simulink model "adaptativeControl"  (R2023b)
settings: Solver=VariableStepAuto  StartTime=0.0  StopTime=time(end)  FixedStep=10e-17  RelTol=1e-3
undefined symbols (not defined in the file): DiscIntNeverNeededParam
libraries: simulink x1
settings Model: Creator=v4pal  LastModifiedBy=v4pal

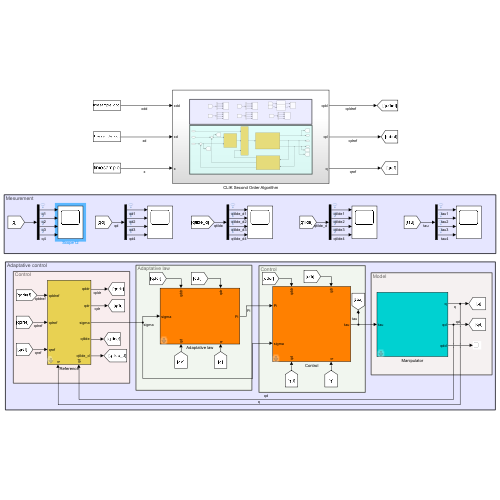
[thumbnail: Simulink's stored preview of the top-level diagram]
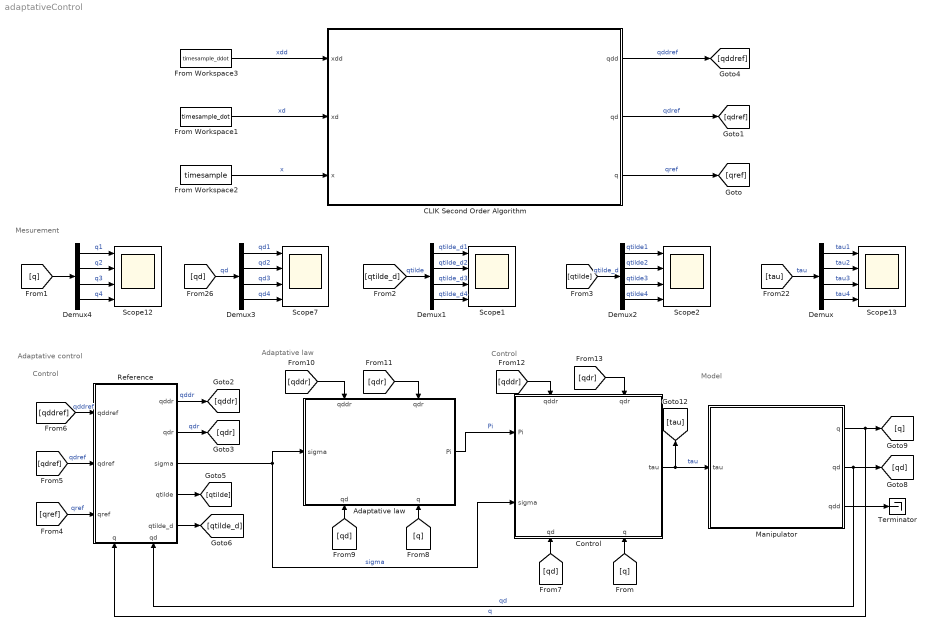
== system adaptativeControl ==
  note: Control
  note: Adaptative law
  note: Mesurement
  note: Control
  note: Adaptative control
  note: Model
  Adaptative law : Subsystem  mask{Kpi=50000}
      mask prompts: Kpi "K_PI"
      settings: PortSchema="{\"entries\":[{\"content\":{\"sides\":[{\"content\":{\"connectorIds\":[\"In1\"]},\"type\":\"ConnectorPlacement.EquallySpacedRectSide\",\"uuid\":\"db15ee83-1f1b-455d-afda-e94c97dcc1f2\"},{\"content\":{\"connectorIds\":[\"Out1\"],\"side\":\"RIGHT\"},\"type\":\"ConnectorPlacement.EquallySpacedRectSide\",\"uuid\":\"41c3f407-56b1-4c5a-b932-c27e17c703ed\"},{\"content\":{\"connectorIds\":[\"In2\",\"In3\"],\"side\":\"TOP\"},\"type\":\"ConnectorPlacement.EquallySpacedRectSide\",\"uuid\":\"e06182f5-78d8-4c0d-9fb3-4a5678e4fb72\"},{\"content\":{\"connectorIds\":[\"In4\",\"In5\"],\"side\":\"BOTTOM\"},\"type\":\"ConnectorPlacement.EquallySpacedRectSide\",\"uuid\":\"7434239a-7bad-433a-9a5d-3d00bbee33a9\"}]},\"type\":\"ConnectorPlacement.EquallySpacedConnector\",\"uuid\":\"7980dd28-bdab-4e8b-a843-8afbd90a57e5\"}],\"packageUris\":[\"http://schema.mathworks.com/mf0/Connector/R2020b\"],\"version\":\"1.0\"}"
  CLIK Second Order Algorithm : Subsystem
  Control : Subsystem  mask{Kd=300}
      settings: PortSchema="{\"entries\":[{\"content\":{\"sides\":[{\"content\":{\"connectorIds\":[\"In1\",\"In2\"]},\"type\":\"ConnectorPlacement.EquallySpacedRectSide\",\"uuid\":\"acb7cdf1-642f-4969-8ed4-672da436f71d\"},{\"content\":{\"connectorIds\":[\"Out1\"],\"side\":\"RIGHT\"},\"type\":\"ConnectorPlacement.EquallySpacedRectSide\",\"uuid\":\"4cc46839-d0fa-4cc4-8f70-8a289b8a20bb\"},{\"content\":{\"connectorIds\":[\"In3\",\"In4\"],\"side\":\"TOP\"},\"type\":\"ConnectorPlacement.EquallySpacedRectSide\",\"uuid\":\"a17c3f60-f42b-40f7-9d43-81c6c657e972\"},{\"content\":{\"connectorIds\":[\"In5\",\"In6\"],\"side\":\"BOTTOM\"},\"type\":\"ConnectorPlacement.EquallySpacedRectSide\",\"uuid\":\"3f3a44a0-a063-4d17-9e5f-328f3f6552e7\"}]},\"type\":\"ConnectorPlacement.EquallySpacedConnector\",\"uuid\":\"f4f2dfd8-ded6-4248-b856-2003e9c40e79\"}],\"packageUris\":[\"http://schema.mathworks.com/mf0/Connector/R2020b\"],\"version\":\"1.0\"}"
  Demux{,1..4} (5 alike) : Demux
  From Workspace1 : FromWorkspace  VariableName=timesample_dot
  From Workspace2 : FromWorkspace  VariableName=timesample
  From Workspace3 : FromWorkspace  VariableName=timesample_ddot
  Manipulator : Subsystem  mask{m_load=4, delta=10}
      mask prompts: m_load "Load Mass [kg]"; delta "Uncertainty [%]"
      mask DialogControl DescGroupVar Prompt: SCARA Dynamic Model
      mask DialogControl DescTextVar Prompt: Scara Dynamic Model with uncertainty and load mass as input.
  Reference : Subsystem  mask{lambda=10}
      settings: PortSchema="{\"entries\":[{\"content\":{\"sides\":[{\"content\":{\"connectorIds\":[\"In1\",\"In2\",\"In3\"]},\"type\":\"ConnectorPlacement.EquallySpacedRectSide\",\"uuid\":\"cb63d9dc-23a2-4ec7-ac11-e398610ef5c2\"},{\"content\":{\"connectorIds\":[\"Out1\",\"Out2\",\"Out3\",\"Out4\",\"Out5\"],\"side\":\"RIGHT\"},\"type\":\"ConnectorPlacement.EquallySpacedRectSide\",\"uuid\":\"29d086a8-0031-4faa-9200-b9934d21fc49\"},{\"content\":{\"side\":\"TOP\"},\"type\":\"ConnectorPlacement.EquallySpacedRectSide\",\"uuid\":\"49ce7692-caef-46fe-903f-68a05e9f5245\"},{\"content\":{\"connectorIds\":[\"In4\",\"In5\"],\"side\":\"BOTTOM\"},\"type\":\"ConnectorPlacement.EquallySpacedRectSide\",\"uuid\":\"32e605e3-ac7e-458a-bf29-966abc0750c1\"}]},\"type\":\"ConnectorPlacement.EquallySpacedConnector\",\"uuid\":\"b951568f-fc90-455a-8420-9594f5316c31\"}],\"packageUris\":[\"http://schema.mathworks.com/mf0/Connector/R2020b\"],\"version\":\"1.0\"}"
  Scope{1..2,7,12..13} (5 alike) : Scope  NumInputPorts=4
  Terminator : Terminator
  wires:
  [qd] -> Demux3/1  "qd"
  Demux2/2 -> Scope2/2  "qtilde2"
  Demux2/3 -> Scope2/3  "qtilde3"
  Demux2/4 -> Scope2/4  "qtilde4"
  [q] -> Demux4/1
  Demux4/4 -> Scope12/4  "q4"
  [qtilde] -> Demux2/1  "qtilde_d"
  Demux1/2 -> Scope1/2  "qtilde_d2"
  Demux1/4 -> Scope1/4  "qtilde_d4"
  [qtilde_d] -> Demux1/1  "qtilde"
  Demux3/4 -> Scope7/4  "qd4"
  Demux3/3 -> Scope7/3  "qd3"
  Demux3/2 -> Scope7/2  "qd2"
  Demux1/1 -> Scope1/1  "qtilde_d1"
  Demux3/1 -> Scope7/1  "qd1"
  Demux/3 -> Scope13/3  "tau3"
  Manipulator/2(qd) -> Reference/5(qd), [qd]  "qd"
  Demux/2 -> Scope13/2  "tau2"
  Control/1(tau) -> Manipulator/1(tau), [tau]  "tau"
  Demux2/1 -> Scope2/1  "qtilde1"
  Demux1/3 -> Scope1/3  "qtilde_d3"
  Demux4/1 -> Scope12/1  "q1"
  Demux/4 -> Scope13/4  "tau4"
  [tau] -> Demux/1  "tau"
  Demux/1 -> Scope13/1  "tau1"
  Demux4/3 -> Scope12/3  "q3"
  Manipulator/3(qdd) -> Terminator/1
  Demux4/2 -> Scope12/2  "q2"
  Manipulator/1(q) -> Reference/4(q), [q]  "q"
  [qddref] -> Reference/1(qddref)  "qddref"
  [qdref] -> Reference/2(qdref)  "qdref"
  [qref] -> Reference/3(qref)  "qref"
  Adaptative law/1(Pi) -> Control/1(Pi)  "Pi"
  Reference/3(sigma) -> Control/2(sigma), Adaptative law/1(sigma)  "sigma"
  [q] -> Control/6(q)
  [qd] -> Control/5(qd)
  [q] -> Adaptative law/5(q)
  [qd] -> Adaptative law/4(qd)
  Reference/1(qddr) -> [qddr]  "qddr"
  Reference/2(qdr) -> [qdr]  "qdr"
  [qddr] -> Adaptative law/2(qddr)
  [qdr] -> Adaptative law/3(qdr)
  [qddr] -> Control/3(qddr)
  [qdr] -> Control/4(qdr)
  Reference/4(qtilde) -> [qtilde]
  Reference/5(qtilde_d) -> [qtilde_d]
  CLIK Second Order Algorithm/2(qd) -> [qdref]  "qdref"
  CLIK Second Order Algorithm/1(qdd) -> [qddref]  "qddref"
  CLIK Second Order Algorithm/3(q) -> [qref]  "qref"
  From Workspace1/1 -> CLIK Second Order Algorithm/2(xd)  "xd"
  From Workspace3/1 -> CLIK Second Order Algorithm/1(xdd)  "xdd"
  From Workspace2/1 -> CLIK Second Order Algorithm/3(x)  "x"

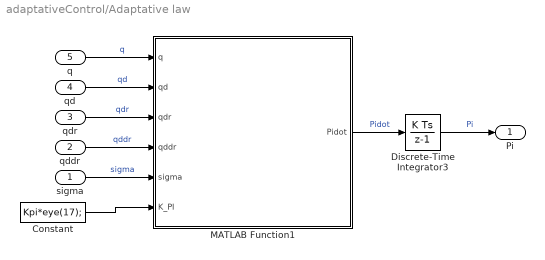
== system adaptativeControl/Adaptative law ==
  sigma : Inport
  qddr : Inport  Port=2
  qdr : Inport  Port=3
  qd : Inport  Port=4
  q : Inport  Port=5
  Constant : Constant  Value=Kpi*eye(17);
  Discrete-Time Integrator3 : DiscreteIntegrator  InitialCondition=[1.2500, 20.0000, 5.0000, 1.2500, 10.0000, 4, 4.000, 4.0000, 1.0000, 0.0100, 0.0100, 0.0050, 0.0010, 0.0001, 0.0001, 0.0100, 0.0050]'  SampleTime=0.001  ICPrevOutput=DiscIntNeverNeededParam  ICPrevScaledInput=DiscIntNeverNeededParam
  MATLAB Function1 : MATLAB Function  TreatAsAtomicUnit=on
  Pi : Outport
  wires:
  q/1 -> MATLAB Function1/1(q)  "q"
  MATLAB Function1/1(Pidot) -> Discrete-Time Integrator3/1  "Pidot"
  Discrete-Time Integrator3/1 -> Pi/1  "Pi"
  qd/1 -> MATLAB Function1/2(qd)  "qd"
  qdr/1 -> MATLAB Function1/3(qdr)  "qdr"
  sigma/1 -> MATLAB Function1/5(sigma)  "sigma"
  qddr/1 -> MATLAB Function1/4(qddr)  "qddr"
  Constant/1 -> MATLAB Function1/6(K_PI)

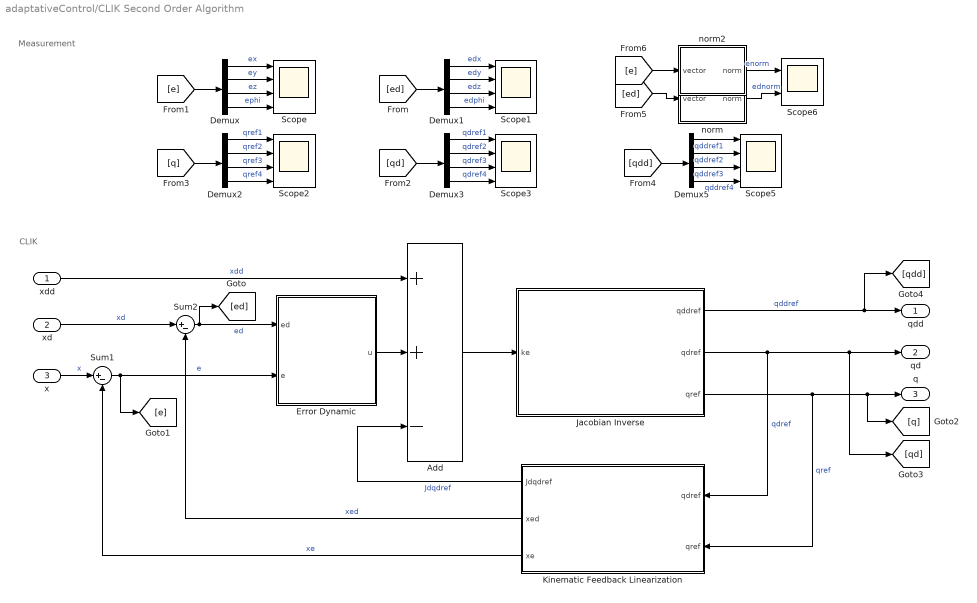
== system adaptativeControl/CLIK Second Order Algorithm ==
  note: CLIK
  note: Measurement
  xdd : Inport
  xd : Inport  Port=2
  x : Inport  Port=3
  Add : Sum  Inputs=++-
  Demux{,1..3,5} (5 alike) : Demux
  Error Dynamic : Subsystem  mask{Kd1=10, Kd2=10, Kd3=10, Kd4=10, Kp1=500, Kp2=500, Kp3=500, Kp4=500, Ki=0}
  Jacobian Inverse : Subsystem
  Kinematic Feedback Linearization : Subsystem
  Scope{,1..3,5} (5 alike) : Scope  NumInputPorts=4
  Scope6 : Scope  NumInputPorts=2
  Sum1 : Sum  Inputs=|+-
  Sum2 : Sum  Inputs=|+-
  norm : Subsystem
  norm2 : Subsystem
  qdd : Outport
  qd : Outport  Port=2
  q : Outport  Port=3
  wires:
  Sum1/1 -> Error Dynamic/2(e), [e]  "e"
  Jacobian Inverse/2(qdref) -> [qd], qd/1, Kinematic Feedback Linearization/1(qdref)  "qdref"
  Sum2/1 -> Error Dynamic/1(ed), [ed]  "ed"
  Add/1 -> Jacobian Inverse/1(ke)
  x/1 -> Sum1/1  "x"
  Jacobian Inverse/3(qref) -> [q], q/1, Kinematic Feedback Linearization/2(qref)  "qref"
  Kinematic Feedback Linearization/1(Jdqdref) -> Add/3  "Jdqdref"
  Kinematic Feedback Linearization/3(xe) -> Sum1/2  "xe"
  Kinematic Feedback Linearization/2(xed) -> Sum2/2  "xed"
  xd/1 -> Sum2/1  "xd"
  Jacobian Inverse/1(qddref) -> [qdd], qdd/1  "qddref"
  xdd/1 -> Add/1  "xdd"
  [ed] -> Demux1/1
  [e] -> Demux/1
  Demux/1 -> Scope/1  "ex"
  Demux/2 -> Scope/2  "ey"
  Demux/3 -> Scope/3  "ez"
  Demux/4 -> Scope/4  "ephi"
  Demux1/1 -> Scope1/1  "edx"
  Demux1/2 -> Scope1/2  "edy"
  Demux1/3 -> Scope1/3  "edz"
  Demux1/4 -> Scope1/4  "edphi"
  Demux3/4 -> Scope3/4  "qdref4"
  Demux3/3 -> Scope3/3  "qdref3"
  Demux3/2 -> Scope3/2  "qdref2"
  Demux3/1 -> Scope3/1  "qdref1"
  Demux2/4 -> Scope2/4  "qref4"
  Demux2/3 -> Scope2/3  "qref3"
  Demux2/2 -> Scope2/2  "qref2"
  Demux2/1 -> Scope2/1  "qref1"
  [q] -> Demux2/1
  [qd] -> Demux3/1
  [qdd] -> Demux5/1
  Demux5/1 -> Scope5/1  "qddref1"
  Demux5/2 -> Scope5/2  "qddref2"
  Demux5/3 -> Scope5/3  "qddref3"
  Demux5/4 -> Scope5/4  "qddref4"
  [e] -> norm2/1(vector)
  norm2/1(norm) -> Scope6/1  "enorm"
  norm/1(norm) -> Scope6/2  "ednorm"
  [ed] -> norm/1(vector)
  Error Dynamic/1(u) -> Add/2

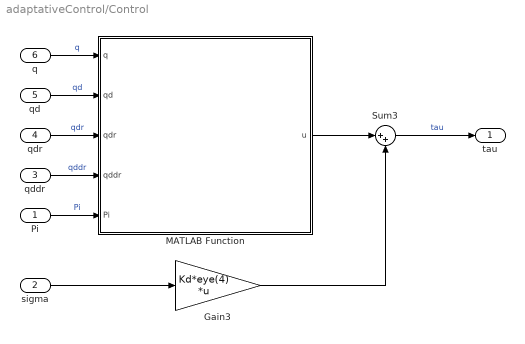
== system adaptativeControl/Control ==
  Pi : Inport
  sigma : Inport  Port=2
  qddr : Inport  Port=3
  qdr : Inport  Port=4
  qd : Inport  Port=5
  q : Inport  Port=6
  Gain3 : Gain  Gain=Kd*eye(4)  Multiplication=Matrix(K*u)
  MATLAB Function : MATLAB Function  TreatAsAtomicUnit=on
  Sum3 : Sum  Inputs=|++
  tau : Outport
  wires:
  Gain3/1 -> Sum3/2
  qd/1 -> MATLAB Function/2(qd)  "qd"
  Pi/1 -> MATLAB Function/5(Pi)  "Pi"
  MATLAB Function/1(u) -> Sum3/1
  Sum3/1 -> tau/1  "tau"
  q/1 -> MATLAB Function/1(q)  "q"
  qdr/1 -> MATLAB Function/3(qdr)  "qdr"
  qddr/1 -> MATLAB Function/4(qddr)  "qddr"
  sigma/1 -> Gain3/1

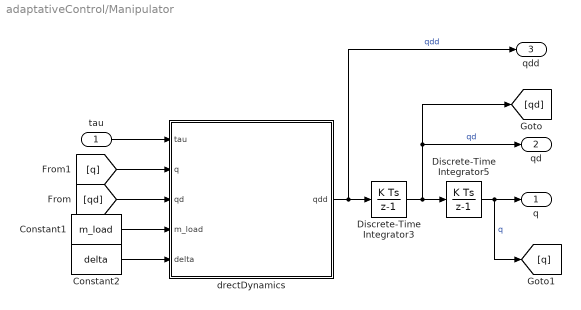
== system adaptativeControl/Manipulator ==
  tau : Inport
  Constant1 : Constant  Value=m_load
  Constant2 : Constant  Value=delta
  Discrete-Time Integrator3 : DiscreteIntegrator  InitialCondition=[0; 0; 0; 0]  SampleTime=0.001  ICPrevOutput=DiscIntNeverNeededParam  ICPrevScaledInput=DiscIntNeverNeededParam
  Discrete-Time Integrator5 : DiscreteIntegrator  InitialCondition=[-1.5706; 0.7851; 0.5000; -0.7855]  SampleTime=0.001  ICPrevOutput=DiscIntNeverNeededParam  ICPrevScaledInput=DiscIntNeverNeededParam
  drectDynamics : MATLAB Function  TreatAsAtomicUnit=on
  q : Outport
  qd : Outport  Port=2
  qdd : Outport  Port=3
  wires:
  tau/1 -> drectDynamics/1(tau)
  Constant1/1 -> drectDynamics/4(m_load)
  drectDynamics/1(qdd) -> qdd/1, Discrete-Time Integrator3/1  "qdd"
  Discrete-Time Integrator3/1 -> [qd], qd/1, Discrete-Time Integrator5/1  "qd"
  Discrete-Time Integrator5/1 -> [q], q/1  "q"
  [qd] -> drectDynamics/3(qd)
  [q] -> drectDynamics/2(q)
  Constant2/1 -> drectDynamics/5(delta)

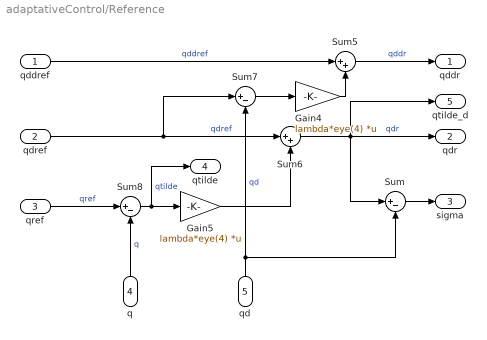
== system adaptativeControl/Reference ==
  qddref : Inport
  qdref : Inport  Port=2
  qref : Inport  Port=3
  q : Inport  Port=4
  qd : Inport  Port=5
  Gain4 : Gain  Gain=lambda*eye(4)  Multiplication=Matrix(K*u)
  Gain5 : Gain  Gain=lambda*eye(4)  Multiplication=Matrix(K*u)
  Sum : Sum  Inputs=|+-
  Sum5 : Sum  Inputs=|++
  Sum6 : Sum  Inputs=|++
  Sum7 : Sum  Inputs=|+-
  Sum8 : Sum  Inputs=|+-
  qddr : Outport
  qdr : Outport  Port=2
  sigma : Outport  Port=3
  qtilde : Outport  Port=4
  qtilde_d : Outport  Port=5
  wires:
  qdref/1 -> Sum7/1, Sum6/1  "qdref"
  Sum8/1 -> qtilde/1, Gain5/1  "qtilde"
  Sum6/1 -> qtilde_d/1, Sum/1, qdr/1  "qdr"
  Gain5/1 -> Sum6/2
  q/1 -> Sum8/2  "q"
  Gain4/1 -> Sum5/2
  Sum7/1 -> Gain4/1
  Sum5/1 -> qddr/1  "qddr"
  qref/1 -> Sum8/1  "qref"
  qddref/1 -> Sum5/1  "qddref"
  qd/1 -> Sum/2, Sum7/2  "qd"
  Sum/1 -> sigma/1

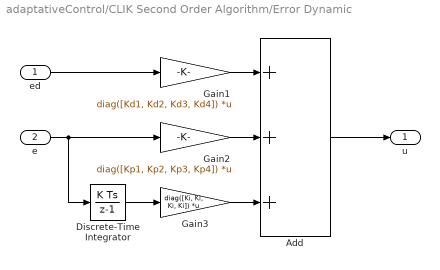
== system adaptativeControl/CLIK Second Order Algorithm/Error Dynamic ==
  ed : Inport
  e : Inport  Port=2
  Add : Sum  Inputs=+++
  Discrete-Time Integrator : DiscreteIntegrator  SampleTime=0.001  ICPrevOutput=DiscIntNeverNeededParam  ICPrevScaledInput=DiscIntNeverNeededParam
  Gain1 : Gain  Gain=diag([Kd1, Kd2, Kd3, Kd4])  Multiplication=Matrix(K*u)
  Gain2 : Gain  Gain=diag([Kp1, Kp2, Kp3, Kp4])  Multiplication=Matrix(K*u)
  Gain3 : Gain  Gain=diag([Ki, Ki, Ki, Ki])  Multiplication=Matrix(K*u)
  u : Outport
  wires:
  Gain2/1 -> Add/2
  Gain1/1 -> Add/1
  ed/1 -> Gain1/1
  e/1 -> Discrete-Time Integrator/1, Gain2/1
  Gain3/1 -> Add/3
  Discrete-Time Integrator/1 -> Gain3/1
  Add/1 -> u/1

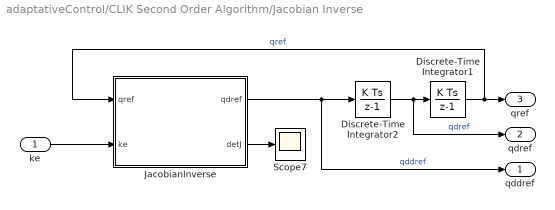
== system adaptativeControl/CLIK Second Order Algorithm/Jacobian Inverse ==
  ke : Inport
  Discrete-Time Integrator1 : DiscreteIntegrator  InitialCondition=[-1.5706; 0.7851; 0.5000; -0.7855]  SampleTime=0.001  ICPrevOutput=DiscIntNeverNeededParam  ICPrevScaledInput=DiscIntNeverNeededParam
  Discrete-Time Integrator2 : DiscreteIntegrator  InitialCondition=[0; 0; 0; 0] %[2.4152; -4.8305; -0.5000; -2.4153]  SampleTime=0.001  ICPrevOutput=DiscIntNeverNeededParam  ICPrevScaledInput=DiscIntNeverNeededParam
  JacobianInverse : MATLAB Function  TreatAsAtomicUnit=on
  Scope7 : Scope
  qddref : Outport
  qdref : Outport  Port=2
  qref : Outport  Port=3
  wires:
  JacobianInverse/2(detJ) -> Scope7/1
  Discrete-Time Integrator2/1 -> qdref/1, Discrete-Time Integrator1/1  "qdref"
  JacobianInverse/1(qdref) -> qddref/1, Discrete-Time Integrator2/1  "qddref"
  Discrete-Time Integrator1/1 -> JacobianInverse/1(qref), qref/1  "qref"
  ke/1 -> JacobianInverse/2(ke)

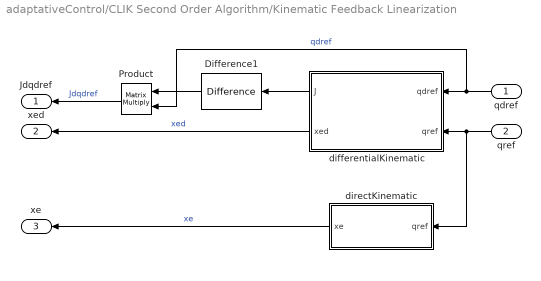
== system adaptativeControl/CLIK Second Order Algorithm/Kinematic Feedback Linearization ==
  qdref : Inport
  qref : Inport  Port=2
  Difference1 : simulink/Discrete/Difference  ICPrevInput=0.0  OutMin=[]  OutMax=[]  OutDataType=fixdt(1, 16)  OutScaling=2^-10  DoSatur=off
  Product : Product  Multiplication=Matrix(*)
  differentialKinematic : MATLAB Function  TreatAsAtomicUnit=on
  directKinematic : MATLAB Function  TreatAsAtomicUnit=on
  Jdqdref : Outport
  xed : Outport  Port=2
  xe : Outport  Port=3
  wires:
  Product/1 -> Jdqdref/1  "Jdqdref"
  Difference1/1 -> Product/1
  qref/1 -> directKinematic/1(qref), differentialKinematic/2(qref)
  differentialKinematic/2(xed) -> xed/1  "xed"
  qdref/1 -> Product/2, differentialKinematic/1(qdref)  "qdref"
  differentialKinematic/1(J) -> Difference1/1
  directKinematic/1(xe) -> xe/1  "xe"

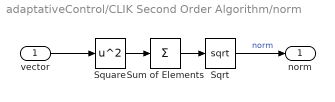
== system adaptativeControl/CLIK Second Order Algorithm/norm ==
  vector : Inport
  Sqrt : Sqrt
  Square : Math  Operator=square
  Sum of Elements : Sum  Inputs=+
  norm : Outport
  wires:
  Sqrt/1 -> norm/1  "norm"
  vector/1 -> Square/1
  Sum of Elements/1 -> Sqrt/1
  Square/1 -> Sum of Elements/1

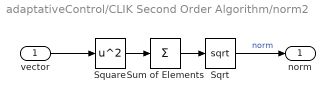
== system adaptativeControl/CLIK Second Order Algorithm/norm2 ==
  vector : Inport
  Sqrt : Sqrt
  Square : Math  Operator=square
  Sum of Elements : Sum  Inputs=+
  norm : Outport
  wires:
  Square/1 -> Sum of Elements/1
  Sum of Elements/1 -> Sqrt/1
  vector/1 -> Square/1
  Sqrt/1 -> norm/1  "norm"

== matlab function adaptativeControl/CLIK Second Order Algorithm/Kinematic Feedback Linearization/differentialKinematic ==
  data: qdref input; J output; qref input; xed output
function [J, xed] = Jacobian(qdref, qref)

    % Init the SCARA manipulator parameters
    a1 = .5; a2 = .5;
    theta1 = qref(1,:); theta2 = qref(2,:);
    
    %% Geometric Jacobian Matrix
    Ja = [-a1*sin(theta1) - a2*sin(theta1 + theta2), - a2*sin(theta1 + theta2), 0, 0;
        a1*cos(theta1) + a2*cos(theta1 + theta2), a2*cos(theta1 + theta2), 0, 0;
        0, 0, -1, 0;
        1, 1, 0, -1;];

    % Vx = Jx1 * qd1 + Jx2 * qd2 +Jx3 * qd3;
    % Vy = Jy1 * qd1 + Jy2 * qd2 +Jy3 * qd3;
    % Vz = Jz1 * qd1 + Jz2 * qd2 +Jz3 * qd3;
    
    %J = Ja(1:3,1:3);
    J = Ja;

    %% Calculation of xe_dot
    xed = J * qdref;

end

== matlab function adaptativeControl/CLIK Second Order Algorithm/Kinematic Feedback Linearization/directKinematic ==
  data: qref input; xe output
function xe = directKinematic(qref)
    
    %% Init the SCARA manipulator parameters and Joint variables
    a1 = .5; a2 = .5; d0 = 1;
    theta1 = qref(1,:); theta2 = qref(2,:); d3 = qref(3,:); theta4 = qref(4,:);

    %% Forward Kinematics link for the SCARA
    k = [a1*cos(theta1) + a2*cos(theta1 + theta2);
        a1*sin(theta1) + a2*sin(theta1 + theta2);
        d0 - d3;
        theta1 + theta2 - theta4;];

    xe = k;

end

== matlab function adaptativeControl/Adaptative law/MATLAB Function1 ==
  data: q input; Pidot output; qd input; qdr input; qddr input; sigma input; K_PI input
function Pidot = regressorTranspose(q,qd,qdr,qddr,sigma,K_PI)

%% Parameter for linear dynamic model
q2 = q(2,:);
qd1 = qd(1,:);
qd2 = qd(2,:);
qdr1 = qdr(1,:);
qdr2 = qdr(2,:);
qdr3 = qdr(3,:);
qdr4 = qdr(4,:);
qddr1 = qddr(1,:);
qddr2 = qddr(2,:);
qddr3 = qddr(3,:); 
qddr4 = qddr(4,:);

a1 = 0.5; a2 = 0.5;
l2 = 0.25;
kr1 = 1; kr2 = 1; kr3 = 50; kr4 = 20;

%% Linear matrix
Y = [qddr1, qddr1*a1^2 + 2*l2*qddr1*cos(q2)*a1, a1*qddr2*cos(q2) - a1*qd1*qdr2*sin(q2) - a1*qd2*qdr1*sin(q2) - a1*qd2*qdr2*sin(q2), qddr1 + qddr2, a1^2*qddr1 + a2^2*qddr1 + a2^2*qddr2 + 2*a1*a2*qddr1*cos(q2) + a1*a2*qddr2*cos(q2) - a1*a2*qd1*qdr2*sin(q2) - a1*a2*qd2*qdr1*sin(q2) - a1*a2*qd2*qdr2*sin(q2), a1^2*qddr1 + a2^2*qddr1 + a2^2*qddr2 + 2*a1*a2*qddr1*cos(q2) + a1*a2*qddr2*cos(q2) - a1*a2*qd1*qdr2*sin(q2) - a1*a2*qd2*qdr1*sin(q2) - a1*a2*qd2*qdr2*sin(q2), qddr1, qddr1 + qddr2, qddr1 + qddr2 - qddr4, kr1^2*qddr1,       qddr1 + kr2*qddr2,           qddr1 + qddr2 + kr3*qddr3,           qddr1 + qddr2 - kr4*qddr4, kr1^2*qdr1,          0,          0,      0;
     0,                                  0,                                             a1*qddr1*cos(q2) + a1*qd1*qdr1*sin(q2), qddr1 + qddr2,                                                                                        a2^2*qddr1 + a2^2*qddr2 + a1*a2*qddr1*cos(q2) + a1*a2*qd1*qdr1*sin(q2),                                                                                        a2^2*qddr1 + a2^2*qddr2 + a1*a2*qddr1*cos(q2) + a1*a2*qd1*qdr1*sin(q2),     0, qddr1 + qddr2, qddr1 + qddr2 - qddr4,           0, qddr2*kr2^2 + qddr1*kr2,           qddr1 + qddr2 + kr3*qddr3,           qddr1 + qddr2 - kr4*qddr4,          0, kr2^2*qdr2,          0,          0;
     0,                                  0,                                                                                  0,             0,                                                                                                                                                qddr3 - 9.8100,                                                                                                                                                qddr3 - 9.8100,     0,             0,                     0,           0,                       0, kr3*qddr1 + kr3*qddr2 + kr3^2*qddr3,                                   0,          0,          0, kr3^2*qdr3,          0;
     0,                                  0,                                                                                  0,             0,                                                                                                                                                             0,                                                                                                                                                             0,     0,             0, qddr4 - qddr2 - qddr1,           0,                       0,                                   0, kr4^2*qddr4 - kr4*qddr2 - kr4*qddr1,          0,          0,          0, kr4^2*qdr4];

%% adaptative law
Pidot = K_PI\(Y')*sigma;

end

== matlab function adaptativeControl/CLIK Second Order Algorithm/Jacobian Inverse/JacobianInverse ==
  data: qref input; ke input; qdref output; detJ output
function [qdref, detJ] = inverseJacobian(qref, ke) % q = [theta1; theta2]

    % Init the SCARA manipulator parameters
    a1 = .5; a2 = .5;

    theta1 = qref(1,:); theta2 = qref(2,:);
    %% Geometric Jacobian Matrix
    J = [-a1*sin(theta1) - a2*sin(theta1 + theta2), - a2*sin(theta1 + theta2), 0, 0;
        a1*cos(theta1) + a2*cos(theta1 + theta2), a2*cos(theta1 + theta2), 0, 0;
        0, 0, -1, 0;
        1, 1, 0, -1;];

    % Vx = Jx1 * qd1 + Jx2 * qd2 +Jx3 * qd3;
    % Vy = Jy1 * qd1 + Jy2 * qd2 +Jy3 * qd3;
    % Vz = Jz1 * qd1 + Jz2 * qd2 +Jz3 * qd3;
    
    %J = J(1:3,1:3);
    
    detJ = det(J);
    % Calculate the inverse of the Jacobian matrix
    J_inv = inv(J);

    % Calculate joint velocities
    qdref = J_inv * ke;

end

== matlab function adaptativeControl/Control/MATLAB Function ==
  data: q input; u output; qd input; qdr input; qddr input; Pi input
function u = regressor(q,qd,qdr,qddr,Pi)

q1 = q(1,:);
q2 = q(2,:);
q3 = q(3,:); 
q4 = q(4,:);
qd1 = qd(1,:);
qd2 = qd(2,:);
qd3 = qd(3,:);
qd4 = qd(4,:);
qdr1 = qdr(1,:);
qdr2 = qdr(2,:);
qdr3 = qdr(3,:);
qdr4 = qdr(4,:);
qddr1 = qddr(1,:);
qddr2 = qddr(2,:);
qddr3 = qddr(3,:);
qddr4 = qddr(4,:);
a1 = 0.5;
a2 = 0.5;

ml1 = 20;
ml2 = 20;
ml3 = 10;
m_load = 4;
Il1 = 4;
Il2 = 4;
Il4 = 1;
Im1 = 0.01;
Im2 = 0.01;
Im3 = 0.005;
Im4 = 0.001;
l1 = 0.25;
l2 = 0.25;
kr1 = 1;
kr2 = 1;
kr3 = 50;
kr4 = 20;
Fm1 =  0.00005;
Fm2 =  0.00005;
Fm3 = 0.01;
Fm4 = 0.005;

Y = [qddr1, qddr1*a1^2 + 2*l2*qddr1*cos(q2)*a1, a1*qddr2*cos(q2) - a1*qd1*qdr2*sin(q2) - a1*qd2*qdr1*sin(q2) - a1*qd2*qdr2*sin(q2), qddr1 + qddr2, a1^2*qddr1 + a2^2*qddr1 + a2^2*qddr2 + 2*a1*a2*qddr1*cos(q2) + a1*a2*qddr2*cos(q2) - a1*a2*qd1*qdr2*sin(q2) - a1*a2*qd2*qdr1*sin(q2) - a1*a2*qd2*qdr2*sin(q2), a1^2*qddr1 + a2^2*qddr1 + a2^2*qddr2 + 2*a1*a2*qddr1*cos(q2) + a1*a2*qddr2*cos(q2) - a1*a2*qd1*qdr2*sin(q2) - a1*a2*qd2*qdr1*sin(q2) - a1*a2*qd2*qdr2*sin(q2), qddr1, qddr1 + qddr2, qddr1 + qddr2 - qddr4, kr1^2*qddr1,       qddr1 + kr2*qddr2,           qddr1 + qddr2 + kr3*qddr3,           qddr1 + qddr2 - kr4*qddr4, kr1^2*qdr1,          0,          0,      0;
     0,                                  0,                                             a1*qddr1*cos(q2) + a1*qd1*qdr1*sin(q2), qddr1 + qddr2,                                                                                        a2^2*qddr1 + a2^2*qddr2 + a1*a2*qddr1*cos(q2) + a1*a2*qd1*qdr1*sin(q2),                                                                                        a2^2*qddr1 + a2^2*qddr2 + a1*a2*qddr1*cos(q2) + a1*a2*qd1*qdr1*sin(q2),     0, qddr1 + qddr2, qddr1 + qddr2 - qddr4,           0, qddr2*kr2^2 + qddr1*kr2,           qddr1 + qddr2 + kr3*qddr3,           qddr1 + qddr2 - kr4*qddr4,          0, kr2^2*qdr2,          0,          0;
     0,                                  0,                                                                                  0,             0,                                                                                                                                                qddr3 - 9.8100,                                                                                                                                                qddr3 - 9.8100,     0,             0,                     0,           0,                       0, kr3*qddr1 + kr3*qddr2 + kr3^2*qddr3,                                   0,          0,          0, kr3^2*qdr3,          0;
     0,                                  0,                                                                                  0,             0,                                                                                                                                                             0,                                                                                                                                                             0,     0,             0, qddr4 - qddr2 - qddr1,           0,                       0,                                   0, kr4^2*qddr4 - kr4*qddr2 - kr4*qddr1,          0,          0,          0, kr4^2*qdr4];
    
u = Y*Pi;
end

== matlab function adaptativeControl/Manipulator/drectDynamics ==
  data: tau input; q input; qdd output; qd input; m_load input; delta input
function qdd = directDynamics(tau,q,qd,m_load,delta)

%% Needed joint position and velocity
q1 = q(1,:);
q2 = q(2,:);
q3 = q(3,:);
qd1 = qd(1,:);
qd2 = qd(2,:);

%% Dynamic Parameters
a1 = 0.5; a2 = 0.5; d0 = 1;
ml1 = 20; ml2 = 20; ml3 = 10;
Il1 = 4; Il2 = 4; Il4 = 1;
Im1 = 0.01; Im2 = 0.01; Im3 = 0.005; Im4 = 0.001;
l1 = 0.25; l2 = 0.25;
kr1 = 1; kr2 = 1; kr3 = 50; kr4 = 20;
Fm1 =  0.00005; Fm2 =  0.00005; Fm3 = 0.01; Fm4 = 0.005;

%% Adding Uncertainty
delta = delta/100; % converting from percentage 
ml1 = ml1 + delta*ml1; ml2 = ml2 + delta*ml2; ml3 = ml3 + delta*ml3;
Il1 = Il1 + delta*Il1; Il2 = Il2 + delta*Il2; Il4 = Il4 + delta*Il4;
l1 = l1 + delta*l1; l2 = l2 + delta*l2;
Fm1 = Fm1 + delta*Fm1;


%% Position vector and z unit vector 
p0 = [0 ; 0 ; d0];
p1 = [a1*cos(q1) ; a1*sin(q1) ; d0];
p2 = [a1*cos(q1) + a2*cos(q1+q2) ; a1*sin(q1) + a2*sin(q1+q2) ; d0];
p3 = p2 - [0 ; 0 ; q3];
p4 = p3;
pl1 = [l1*cos(q1) ; l1*sin(q1) ; d0];
pl2 = [a1*cos(q1) + l2*cos(q1+q2) ; a1*sin(q1) + l2*sin(q1+q2) ; d0];
pl3 = p3; % ????
pl4 = p4; % 
z0 = [0 0 1]';
z1 = [0 0 1]';
z2 = [0 0 -1]';
z3 = [0 0 -1]';

%% Positional and orientation jacobian of links (JPl JOl JOm)
JP_l1 = [cross(z0,pl1-p0) zeros(3,3)];
JP_l2 = [cross(z0,pl2-p0) cross(z1,pl2-p1) zeros(3,2)];
JP_l3 = [cross(z0,pl3-p0) cross(z1,pl3-p1) z2 zeros(3,1)]; 
JP_l4 = [cross(z0,pl4-p0) cross(z1,pl4-p1) z2 cross(z3,pl4-p3)]; %m4=mload

JO_l1 = [z0 zeros(3,3)];
JO_l2 = [z0 z1 zeros(3,2)];
%JO_l3 = [z0 z1 zeros(3,2)]; Il3=0
JO_l4 = [z0 z1 zeros(3,1) z3];

%assuming zm1=z0, zm2=z1, zm3=-z2, zm4=z3-->it's on the joint
JO_m1 = JO_l1;
JO_m1(:,1) = kr1*z0;
JO_m2 = JO_l2;  
JO_m2(:,2) = kr2*z1;
JO_m3 = [z0 z1 zeros(3,2)]; 
JO_m3(:,3) = kr3*z2;
JO_m4 = JO_l4;
JO_m4(:,4) = kr4*z3;

%% Inertia matrix B (eq 7.32)
B1 = ml1*(JP_l1'*JP_l1) + Il1*(JO_l1'*JO_l1) + Im1*(JO_m1'*JO_m1) ; 
B2 = ml2*(JP_l2'*JP_l2) + Il2*(JO_l2'*JO_l2) + Im2*(JO_m2'*JO_m2) ; 
B3 = ml3*(JP_l3'*JP_l3) + 0 + Im3*(JO_m3'*JO_m3) ; %Il3=0
B4 = m_load*(JP_l4'*JP_l4) + Il4*(JO_l4'*JO_l4) + Im4*(JO_m4'*JO_m4) ; 
B = B1 + B2 + B3 + B4;

%% Gravity forces(Formula 7.39)
g0 = [0 0 -9.81]';
g1 = - (ml1*g0'*JP_l1(:,1) + ml2*g0'*JP_l2(:,1) + ml3*g0'*JP_l3(:,1) + m_load*g0'*JP_l4(:,1));
g2 = - (ml1*g0'*JP_l1(:,2) + ml2*g0'*JP_l2(:,2) + ml3*g0'*JP_l3(:,2) + m_load*g0'*JP_l4(:,2));
g3 = - (ml1*g0'*JP_l1(:,3) + ml2*g0'*JP_l2(:,3) + ml3*g0'*JP_l3(:,3) + m_load*g0'*JP_l4(:,3));
g4 = - (ml1*g0'*JP_l1(:,4) + ml2*g0'*JP_l2(:,4) + ml3*g0'*JP_l3(:,4) + m_load*g0'*JP_l4(:,4));
g = [g1 g2 g3 g4]';

%% Coriolis matrix C
C = [-a1*qd2*sin(q2)*(a2*m_load + a2*ml3 + l2*ml2), -a1*sin(q2)*(qd1 + qd2)*(a2*m_load + a2*ml3 + l2*ml2), 0, 0;
      a1*qd1*sin(q2)*(a2*m_load + a2*ml3 + l2*ml2),  0, 0, 0;
      0, 0, 0, 0;
      0, 0, 0, 0]; 

%% Friction
Fv = diag([kr1^2*Fm1 kr2^2*Fm2 kr3^2*Fm3 kr4^2*Fm4]);

%% Acceleration computation
qdd = inv(B)*(tau - C*qd -Fv*qd -g);

end
